simulink model "FunctionControl"  (R2023a)
settings: Solver=VariableStepAuto  StartTime=0.0  StopTime=10.0  RelTol=1e-3
settings Model: Creator=aan18022  LastModifiedBy=COMPUTER

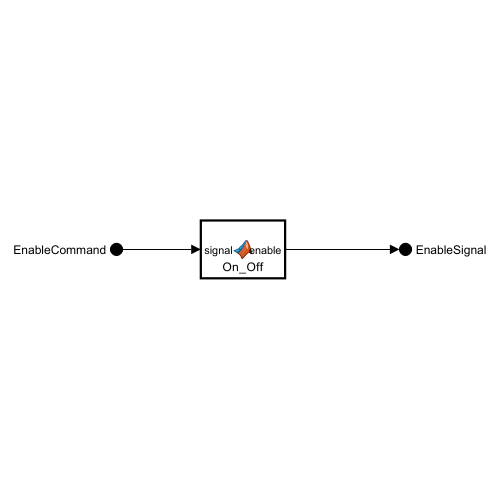
[thumbnail: Simulink's stored preview of the top-level diagram]
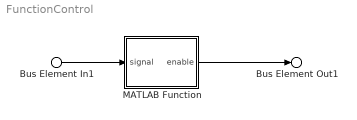
== system FunctionControl ==
  Bus Element In1 : Inport  PortName=EnableCommand
  MATLAB Function : MATLAB Function  TreatAsAtomicUnit=on
  Bus Element Out1 : Outport  PortName=EnableSignal
  wires:
  Bus Element In1/1 -> MATLAB Function/1(signal)
  MATLAB Function/1(enable) -> Bus Element Out1/1

== matlab function FunctionControl/MATLAB Function ==
  data: enable output; signal input
function enable = On_Off(signal)

if signal == 1
    enable = 1;
else
    enable = 0;
end
